simulink model "SimulinkschaltbildTeil2"  (R2014b)
settings: Solver=ode45  StartTime=0.0  StopTime=10.0  RelTol=1e-3
settings Model: Creator=Florian  LastModifiedBy=Florian

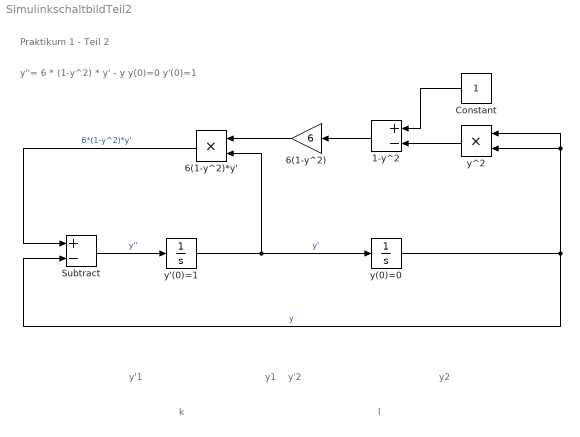
== system SimulinkschaltbildTeil2 ==
  note: l
  note: k
  note: y1
  note: y2
  note: y'2
  note: y'1
  note: Praktikum 1 - Teil 2
  note: y''= 6 * (1-y^2) * y' - y y(0)=0 y'(0)=1
  1-y^2 : Sum  Inputs=+-
  6(1-y^2) : Gain  Gain=6
  6(1-y^2)*y' : Product
  Constant : Constant
  Subtract : Sum  Inputs=+-
  y'(0)=1 : Integrator
  y(0)=0 : Integrator
  y^2 : Product
  wires:
  y'(0)=1/1 -> 6(1-y^2)*y'/2, y(0)=0/1  "y'"
  Subtract/1 -> y'(0)=1/1  "y''"
  y(0)=0/1 -> Subtract/2, y^2/2, y^2/1  "y"
  y^2/1 -> 1-y^2/2
  1-y^2/1 -> 6(1-y^2)/1
  6(1-y^2)/1 -> 6(1-y^2)*y'/1
  6(1-y^2)*y'/1 -> Subtract/1  "6*(1-y^2)*y'"
  Constant/1 -> 1-y^2/1
